simulink model "quad_simulation_with_linearization_around_wrench"  (R2018b)
settings: Solver=ode45  StartTime=0.0  StopTime=30  FixedStep=0.001  MaxStep=0.001  MinStep=0.0001  RelTol=1e-3
values from neighbouring files (symbols this model uses):
  b = 7e-9    (= 7e-09)    [Controller_Calc_W.m]    (also in Controller_Calc_Wrench.m; SDFO.m = parameters(7); SDR.m = parameters(7); hjb_minimum_fuel_continuous_time.m = parameters(7))
  g = 9.8    [Controller_Calc_W.m]    (also in Controller_Calc_Wrench.m; SDFO.m = parameters(12); SDR.m = parameters(12); hjb_minimum_fuel_continuous_time.m = parameters(12))
  Ixx = 2.661e-5    (= 2.661e-05)    [Controller_Calc_W.m]    (also in Controller_Calc_Wrench.m; SDFO.m = parameters(2); SDR.m = parameters(2); hjb_minimum_fuel_continuous_time.m = parameters(2))
  Iyy = 2.661e-5    (= 2.661e-05)    [Controller_Calc_W.m]    (also in Controller_Calc_Wrench.m; SDFO.m = parameters(3); SDR.m = parameters(3); hjb_minimum_fuel_continuous_time.m = parameters(3))
  Izz = 2.661e-5    (= 2.661e-05)    [Controller_Calc_W.m]    (also in Controller_Calc_Wrench.m; SDFO.m = parameters(4); SDR.m = parameters(4); hjb_minimum_fuel_continuous_time.m = parameters(4))
  k = 2e-6    (= 2e-06)    [Controller_Calc_W.m]    (also in Controller_Calc_Wrench.m; SDFO.m = parameters(5); SDR.m = parameters(5); hjb_minimum_fuel_continuous_time.m = parameters(5))
  K = zeros(4, 12, N)    [hjb_minimum_fuel_continuous_time.m]    (also in hjb_minimum_fuel_discrete_time.m)
  kd = 0    [Controller_Calc_W.m]    (also in Controller_Calc_Wrench.m; SDFO.m = parameters(8); SDR.m = parameters(8); hjb_minimum_fuel_continuous_time.m = parameters(8))
  L = 0.035    [Controller_Calc_W.m]    (also in Controller_Calc_Wrench.m; SDFO.m = parameters(6); SDR.m = parameters(6); hjb_minimum_fuel_continuous_time.m = parameters(6))
  m = w .* sign(w)    [SDFO.m]    (also in SDR.m = (u + ones(4, 1) * mq * g / 4); hjb_regulation_continuous_time.m = (u(:, i) + ones(4, 1) * mq * g / 4); hjb_regulation_discrete_time.m = (u(:, i) + ones(4, 1) * mq * g / 4))
  mq = 0.3812    [Controller_Calc_W.m]    (also in Controller_Calc_Wrench.m; SDFO.m = parameters(1); SDR.m = parameters(1); hjb_minimum_fuel_continuous_time.m = parameters(1))
  N = numel(t)    [Controller_Calc_W.m]    (also in Controller_Calc_Wrench.m; SDFO.m; SDR.m; hjb_minimum_fuel_continuous_time.m)
  r = 0.03    [Controller_Calc_W.m]    (also in Controller_Calc_Wrench.m; SDFO.m = parameters(10); SDR.m = parameters(10); hjb_minimum_fuel_continuous_time.m = parameters(10))
  rho = 0.037    [Controller_Calc_W.m]    (also in Controller_Calc_Wrench.m; SDFO.m = parameters(9); SDR.m = parameters(9); hjb_minimum_fuel_continuous_time.m = parameters(9))
  xd = 2    [Controller_Calc_W.m]    (also in Controller_Calc_Wrench.m; SDFO.m; SDR.m; hjb_minimum_fuel_continuous_time.m)
  yd = 2    [Controller_Calc_W.m]    (also in Controller_Calc_Wrench.m; SDFO.m; SDR.m; hjb_minimum_fuel_continuous_time.m)
  z_offset = 0.02    [Controller_Calc_W.m]    (also in Controller_Calc_Wrench.m; SDFO.m = parameters(11); SDR.m = parameters(11); hjb_minimum_fuel_continuous_time.m = parameters(11))
  zd = 1    [Controller_Calc_W.m]    (also in Controller_Calc_Wrench.m; SDFO.m; SDR.m; hjb_minimum_fuel_continuous_time.m)
undefined symbols (not defined in the file or in its folder): X, Y, Z
libraries: sm_lib x31, nesl_utility x15
settings Model: Creator=farid  LastModifiedBy=farid
settings SolverCC: ShapePreserveControl=EnableAll
settings DebuggingCC: IgnoredZcDiagnostic=none
settings ExplorerConfigSet: InternalSimMechanicsExplorerSettings="<ExplorerConfiguration><canonicalview>default</canonicalview><AnimationSetting><BasePlaybackSpeed>1.0</BasePlaybackSpeed><PlaybackSpeedFactor>1.0</PlaybackSpeedFactor></AnimationSetting><TilePanel><TileInfo><Tiles Columns=\"1\" Count=\"1\" Rows=\"1\"><Column Weight=\"1\"/><Row Weight=\"1\"/><Tile Height=\"1\" Width=\"1\" X=\"0\" Y=\"0\"/></Tiles></TileInfo><SceneInfo><SceneViewer><BGColor><R>0.60000002384185791</R><G>0.60000002384185791</G><B>0.60000002384185791</B></BGColor><Camera><DoPerspective>on</DoPerspective><Position><X>3.33949980158925674</X><Y>0.311821910931282698</Y><Z>2.70298018653747674</Z></Position><Center><X>1.08899615373952652</X><Y>1.13154056192934438</Y><Z>1.11569979798405505</Z></Center><Up><X>-0.544111387688414605</X><Y>0.115372635576885818</Y><Z>0.831042690087477443</Z></Up><ViewLimDist>1</ViewLimDist><YLim>0.466307658154998583</YLim><XLim>0.669757770788069529</XLim></Camera></SceneViewer></SceneInfo></TilePanel><MechEditorPanel><Cameras><Camera><Id>Camera1</Id><Value><Name>Camera1</Name><NativeCamera><PositionKeyframeSet/><CenterKeyframeSet/><UpVectorKeyframeSet/></NativeCamera></Value></Camera></Cameras><GfxPanelCameraMap><MapElement CameraMLId=\"Camera1\" GfxPanelIndex=\"0\"/></GfxPanelCameraMap><VideoCreator><PlaybackSpeedRatio>1.0</PlaybackSpeedRatio><FrameRate>60</FrameRate><VideoFormat>Motion JPEG AVI</VideoFormat><FrameSize>[1280 720]</FrameSize></VideoCreator></MechEditorPanel></ExplorerConfiguration>"

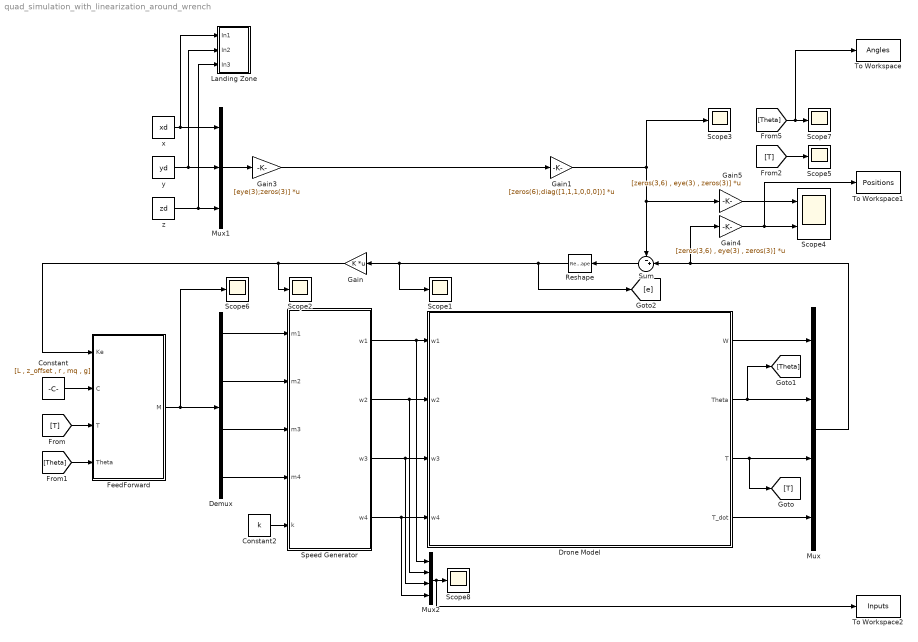
== system quad_simulation_with_linearization_around_wrench ==
  Constant : Constant  Value=[L , z_offset , r , mq , g]
  Constant2 : Constant  Value=k
  Demux : Demux
  Drone Model : Subsystem  mask{mq=mq, Ixx=Ixx, Iyy=Iyy, Izz=Izz, k=k, L=L, b=b, kd=kd, rho=rho, r=r, z_offset=z_offset, g=g}
      mask prompts: z_offset "offset in z:"
  FeedForward : MATLAB Function  TreatAsAtomicUnit=on
  Gain : Gain  Gain=K  Multiplication=Matrix(K*u) (u vector)
  Gain1 : Gain  Gain=[zeros(6);diag([1,1,1,0,0,0])]  Multiplication=Matrix(K*u) (u vector)
  Gain3 : Gain  Gain=[eye(3);zeros(3)]  Multiplication=Matrix(K*u) (u vector)
  Gain4 : Gain  Gain=[zeros(3,6) , eye(3) , zeros(3)]  Multiplication=Matrix(K*u) (u vector)
  Gain5 : Gain  Gain=[zeros(3,6) , eye(3) , zeros(3)]  Multiplication=Matrix(K*u) (u vector)
  Landing Zone : Subsystem
  Mux : Mux
  Mux1 : Mux  Inputs=3
  Mux2 : Mux
  Reshape : Reshape  OutputDimensionality=Column vector (2-D)
  Scope{1..3,5..8} (7 alike) : Scope
  Scope4 : Scope  NumInputPorts=2
  Speed Generator : MATLAB Function  TreatAsAtomicUnit=on
  Sum : Sum  Inputs=-+|
  To Workspace : ToWorkspace  VariableName=Angles  SaveFormat=Timeseries  SampleTime=-1
  To Workspace1 : ToWorkspace  VariableName=Positions  SaveFormat=Timeseries  SampleTime=-1
  To Workspace2 : ToWorkspace  VariableName=Inputs  SaveFormat=Timeseries  SampleTime=-1
  x : Constant  Value=xd
  y : Constant  Value=yd
  z : Constant  Value=zd
  wires:
  Speed Generator/1(w1) -> Mux2/1, Drone Model/1(w1)
  Speed Generator/2(w2) -> Mux2/2, Drone Model/2(w2)
  Speed Generator/3(w3) -> Mux2/3, Drone Model/3(w3)
  Speed Generator/4(w4) -> Mux2/4, Drone Model/4(w4)
  Drone Model/1(W) -> Mux/1
  Drone Model/2(Theta) -> [Theta], Mux/2
  Drone Model/3(T) -> [T], Mux/3
  Drone Model/4(T_dot) -> Mux/4
  Demux/1 -> Speed Generator/1(m1)
  Demux/2 -> Speed Generator/2(m2)
  Demux/3 -> Speed Generator/3(m3)
  Demux/4 -> Speed Generator/4(m4)
  Mux1/1 -> Gain3/1
  Mux/1 -> Gain4/1, Sum/2
  Gain3/1 -> Gain1/1
  Gain5/1 -> Scope4/1
  Gain4/1 -> To Workspace1/1, Scope4/2
  Gain1/1 -> Sum/1, Gain5/1, Scope3/1
  x/1 -> Landing Zone/1(In1), Mux1/1
  z/1 -> Landing Zone/3(In3), Mux1/3
  y/1 -> Landing Zone/2(In2), Mux1/2
  FeedForward/1(M) -> Scope6/1, Demux/1
  [T] -> FeedForward/3(T)
  [Theta] -> FeedForward/4(Theta)
  Constant/1 -> FeedForward/2(C)
  Sum/1 -> Reshape/1
  Reshape/1 -> [e], Gain/1, Scope1/1
  Gain/1 -> FeedForward/1(Ke), Scope2/1
  Constant2/1 -> Speed Generator/5(k)
  [Theta] -> To Workspace/1, Scope7/1
  [T] -> Scope5/1
  Mux2/1 -> To Workspace2/1, Scope8/1

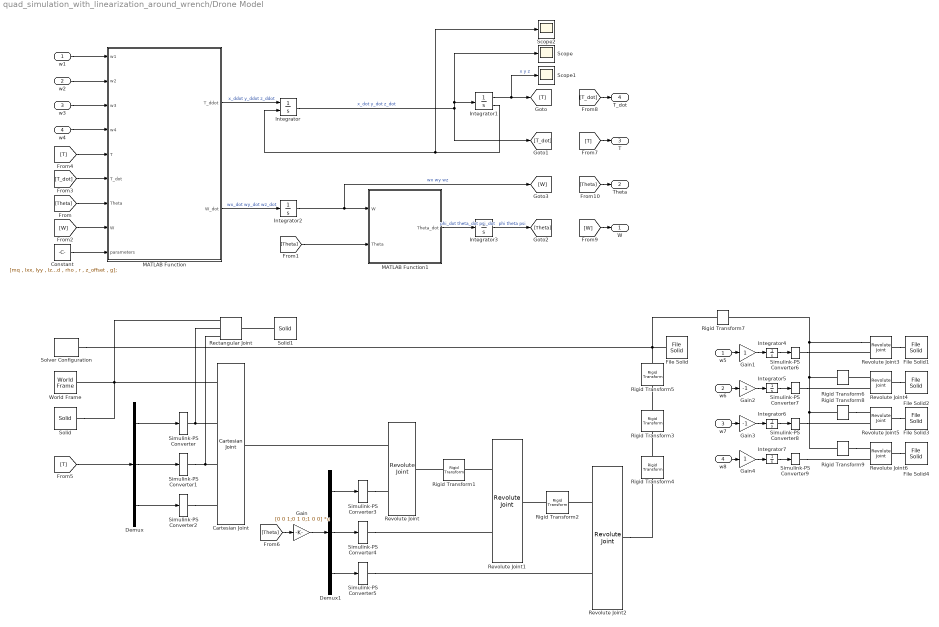
== system quad_simulation_with_linearization_around_wrench/Drone Model ==
  w1 : Inport
  w2 : Inport  Port=2
  w3 : Inport  Port=3
  w4 : Inport  Port=4
  Cartesian Joint : sm_lib/Joints/Cartesian Joint  SenseConstraintForce=off  SenseConstraintForceX=off  SenseConstraintForceY=off  SenseConstraintForceZ=off  SenseConstraintTorque=off  SenseConstraintTorqueX=off  SenseConstraintTorqueY=off  SenseConstraintTorqueZ=off  SenseTotalForce=off  SenseTotalForceX=off  SenseTotalForceY=off  SenseTotalForceZ=off  SenseTotalTorque=off  SenseTotalTorqueX=off  SenseTotalTorqueY=off  SenseTotalTorqueZ=off  CompositeWrenchDir=FollowerOnBase  CompositeWrenchFrame=BaseFrame  PxEquilibriumPosition=0  PxEquilibriumPositionUnits=m  PxSpringStiffness=0  PxSpringStiffnessUnits=N/m  PxDampingCoefficient=0  PxDampingCoefficientUnits=N/(m/s)  PxTorqueActuationMode=ComputedTorque  PxMotionActuationMode=InputMotion  PxSensePosition=off  PxSenseVelocity=off  PxSenseAcceleration=off  PxSenseTorqueForce=off  PxPositionTargetSpecify=off  PxPositionTargetPriority=High  PxPositionTargetValue=0  PxPositionTargetValueUnits=m  PxVelocityTargetSpecify=off  PxVelocityTargetPriority=High  PxVelocityTargetValue=0  PxVelocityTargetValueUnits=m/s  PyEquilibriumPosition=0  PyEquilibriumPositionUnits=m  PySpringStiffness=0  PySpringStiffnessUnits=N/m  PyDampingCoefficient=0  PyDampingCoefficientUnits=N/(m/s)  PyTorqueActuationMode=ComputedTorque  PyMotionActuationMode=InputMotion  PySensePosition=off  PySenseVelocity=off  PySenseAcceleration=off  PySenseTorqueForce=off  PyPositionTargetSpecify=off  PyPositionTargetPriority=High  PyPositionTargetValue=0  PyPositionTargetValueUnits=m  PyVelocityTargetSpecify=off  PyVelocityTargetPriority=High  PyVelocityTargetValue=0  PyVelocityTargetValueUnits=m/s  PzEquilibriumPosition=0  PzEquilibriumPositionUnits=m  PzSpringStiffness=0  PzSpringStiffnessUnits=N/m  PzDampingCoefficient=0  PzDampingCoefficientUnits=N/(m/s)  PzTorqueActuationMode=ComputedTorque  PzMotionActuationMode=InputMotion  PzSensePosition=off  PzSenseVelocity=off  PzSenseAcceleration=off  PzSenseTorqueForce=off  PzPositionTargetSpecify=on  PzPositionTargetPriority=High  PzPositionTargetValue=1  PzPositionTargetValueUnits=m  PzVelocityTargetSpecify=off  PzVelocityTargetPriority=High  PzVelocityTargetValue=0  PzVelocityTargetValueUnits=m/s
  Constant : Constant  Value=[mq , Ixx, Iyy , Izz , k , L , b , kd , rho , r , z_offset , g];
  Demux : Demux  Outputs=3
  Demux1 : Demux  Outputs=3
  File Solid : sm_lib/Body Elements/File Solid  ExtGeomFileName=/mnt/HDD Disk/Documents/MATLAB/Sahar Nasimi Nejad/dron.stl  UnitType=Custom  ExtGeomFileUnits=mm  InertiaType=Custom  Mass=1  MassUnits=kg  CenterOfMass=[0 0 0]  CenterOfMassUnits=m  MomentsOfInertia=[1 1 1]  MomentsOfInertiaUnits=kg*m^2  ProductsOfInertia=[0 0 0]  ProductsOfInertiaUnits=kg*m^2  BasedOnType=Density  Density=2  DensityUnits=g/cm^3  DoExposeReferenceFrame=on  SerializedFrames=<Frames/>  GraphicType=FromGeometry  MarkerShape=Sphere  MarkerSize=10  GraphicVisPropType=SimpleVisualProperties  GraphicDiffuseColor=[0.2 0.8 0.0]  GraphicSpecularColor=[0.5 0.5 0.5 1.0]  GraphicAmbientColor=[0.15 0.15 0.15 1.0]  GraphicEmissiveColor=[0.0 0.0 0.0 1.0]  GraphicShininess=75  GraphicOpacity=1.0
  File Solid{1..4} (4 alike) : sm_lib/Body Elements/File Solid  ExtGeomFileName=/mnt/HDD Disk/Documents/MATLAB/Optimal Control/propeller.stl  UnitType=Custom  ExtGeomFileUnits=mm  InertiaType=Custom  Mass=1  MassUnits=kg  CenterOfMass=[0 0 0]  CenterOfMassUnits=m  MomentsOfInertia=[1 1 1]  MomentsOfInertiaUnits=kg*m^2  ProductsOfInertia=[0 0 0]  ProductsOfInertiaUnits=kg*m^2  BasedOnType=Density  Density=2  DensityUnits=g/cm^3  DoExposeReferenceFrame=on  SerializedFrames=<Frames/>  GraphicType=FromGeometry  MarkerShape=Sphere  MarkerSize=10  GraphicVisPropType=SimpleVisualProperties  GraphicDiffuseColor=[1.0 1.0 0.0]  GraphicSpecularColor=[0.5 0.5 0.5 1.0]  GraphicAmbientColor=[0.15 0.15 0.15 1.0]  GraphicEmissiveColor=[0.0 0.0 0.0 1.0]  GraphicShininess=75  GraphicOpacity=1.0
  Gain : Gain  Gain=[0 0 1;0 1 0;1 0 0]  Multiplication=Matrix(K*u)
  Gain1 : Gain
  Gain2 : Gain  Gain=-1
  Gain3 : Gain  Gain=-1
  Gain4 : Gain
  Integrator : Integrator  ExternalReset=either  InitialCondition=[0;0;0]
  Integrator1 : Integrator  InitialCondition=[0;0;1]  LimitOutput=on  UpperSaturationLimit=[inf;inf;inf]  LowerSaturationLimit=[-inf;-inf;0]  ShowSaturationPort=on
  Integrator2 : Integrator  InitialCondition=[0;0;0]
  Integrator3 : Integrator  InitialCondition=[0;0;0]
  Integrator{4..7} (4 alike) : Integrator
  MATLAB Function : MATLAB Function  TreatAsAtomicUnit=on
  MATLAB Function1 : MATLAB Function  TreatAsAtomicUnit=on
  Rectangular Joint : sm_lib/Joints/Rectangular Joint  SenseConstraintForce=off  SenseConstraintForceX=off  SenseConstraintForceY=off  SenseConstraintForceZ=off  SenseConstraintTorque=off  SenseConstraintTorqueX=off  SenseConstraintTorqueY=off  SenseConstraintTorqueZ=off  SenseTotalForce=off  SenseTotalForceX=off  SenseTotalForceY=off  SenseTotalForceZ=off  SenseTotalTorque=off  SenseTotalTorqueX=off  SenseTotalTorqueY=off  SenseTotalTorqueZ=off  CompositeWrenchDir=FollowerOnBase  CompositeWrenchFrame=BaseFrame  PxEquilibriumPosition=0  PxEquilibriumPositionUnits=m  PxSpringStiffness=0  PxSpringStiffnessUnits=N/m  PxDampingCoefficient=0  PxDampingCoefficientUnits=N/(m/s)  PxTorqueActuationMode=ComputedTorque  PxMotionActuationMode=InputMotion  PxSensePosition=off  PxSenseVelocity=off  PxSenseAcceleration=off  PxSenseTorqueForce=off  PxPositionTargetSpecify=off  PxPositionTargetPriority=High  PxPositionTargetValue=0  PxPositionTargetValueUnits=m  PxVelocityTargetSpecify=off  PxVelocityTargetPriority=High  PxVelocityTargetValue=0  PxVelocityTargetValueUnits=m/s  PyEquilibriumPosition=0  PyEquilibriumPositionUnits=m  PySpringStiffness=0  PySpringStiffnessUnits=N/m  PyDampingCoefficient=0  PyDampingCoefficientUnits=N/(m/s)  PyTorqueActuationMode=ComputedTorque  PyMotionActuationMode=InputMotion  PySensePosition=off  PySenseVelocity=off  PySenseAcceleration=off  PySenseTorqueForce=off  PyPositionTargetSpecify=off  PyPositionTargetPriority=High  PyPositionTargetValue=0  PyPositionTargetValueUnits=m  PyVelocityTargetSpecify=off  PyVelocityTargetPriority=High  PyVelocityTargetValue=0  PyVelocityTargetValueUnits=m/s
      settings: SourceProductName=Simscape Multibody
  Revolute Joint{,1..6} (7 alike) : sm_lib/Joints/Revolute Joint  SenseConstraintForce=off  SenseConstraintForceX=off  SenseConstraintForceY=off  SenseConstraintForceZ=off  SenseConstraintTorque=off  SenseConstraintTorqueX=off  SenseConstraintTorqueY=off  SenseConstraintTorqueZ=off  SenseTotalForce=off  SenseTotalForceX=off  SenseTotalForceY=off  SenseTotalForceZ=off  SenseTotalTorque=off  SenseTotalTorqueX=off  SenseTotalTorqueY=off  SenseTotalTorqueZ=off  CompositeWrenchDir=FollowerOnBase  CompositeWrenchFrame=BaseFrame  EquilibriumPosition=0  EquilibriumPositionUnits=deg  SpringStiffness=0  SpringStiffnessUnits=N*m/deg  DampingCoefficient=0  DampingCoefficientUnits=N*m/(deg/s)  TorqueActuationMode=ComputedTorque  MotionActuationMode=InputMotion  SensePosition=off  SenseVelocity=off  SenseAcceleration=off  SenseTorqueForce=off  PositionTargetSpecify=off  PositionTargetPriority=High  PositionTargetValue=0  PositionTargetValueUnits=deg  VelocityTargetSpecify=off  VelocityTargetPriority=High  VelocityTargetValue=0  VelocityTargetValueUnits=deg/s
  Rigid Transform1 : sm_lib/Frames and Transforms/Rigid Transform  TranslationMethod=None  TranslationStandardOffset=0  TranslationLengthUnit=m  TranslationStandardAxis=+Z  TranslationCartesianOffset=[0 0 0]  TranslationROffset=0  TranslationROffsetUnits=m  TranslationZOffset=0  TranslationZOffsetUnits=m  TranslationThetaOffset=0  TranslationThetaOffsetUnits=deg  RotationMethod=StandardAxis  RotationAngleUnits=deg  RotationStandardAxis=-X  RotationAngle=90  RotationArbitraryAxis=[0 0 1]  FollAlignAxisA=+X  BaseAlignAxisA=+Y  FollAlignAxisB=+Y  BaseAlignAxisB=+Z  RotationSequenceAxes=FollowerAxes  RotationSequence=XYX  RotationSequenceAngles=[0 0 0]  RotationSequenceAnglesUnits=deg  RotationMatrix=[1 0 0; 0 1 0; 0 0 1]
  Rigid Transform2 : sm_lib/Frames and Transforms/Rigid Transform  TranslationMethod=None  TranslationStandardOffset=0  TranslationLengthUnit=m  TranslationStandardAxis=+Z  TranslationCartesianOffset=[0 0 0]  TranslationROffset=0  TranslationROffsetUnits=m  TranslationZOffset=0  TranslationZOffsetUnits=m  TranslationThetaOffset=0  TranslationThetaOffsetUnits=deg  RotationMethod=StandardAxis  RotationAngleUnits=deg  RotationStandardAxis=+Y  RotationAngle=90  RotationArbitraryAxis=[0 0 1]  FollAlignAxisA=+X  BaseAlignAxisA=+Y  FollAlignAxisB=+Y  BaseAlignAxisB=+Z  RotationSequenceAxes=FollowerAxes  RotationSequence=XYX  RotationSequenceAngles=[0 0 0]  RotationSequenceAnglesUnits=deg  RotationMatrix=[1 0 0; 0 1 0; 0 0 1]
  Rigid Transform3 : sm_lib/Frames and Transforms/Rigid Transform  TranslationMethod=None  TranslationStandardOffset=0  TranslationLengthUnit=m  TranslationStandardAxis=+Z  TranslationCartesianOffset=[0 0 0]  TranslationROffset=0  TranslationROffsetUnits=m  TranslationZOffset=0  TranslationZOffsetUnits=m  TranslationThetaOffset=0  TranslationThetaOffsetUnits=deg  RotationMethod=StandardAxis  RotationAngleUnits=deg  RotationStandardAxis=+X  RotationAngle=90  RotationArbitraryAxis=[0 0 1]  FollAlignAxisA=+X  BaseAlignAxisA=+Y  FollAlignAxisB=+Y  BaseAlignAxisB=+Z  RotationSequenceAxes=FollowerAxes  RotationSequence=XYX  RotationSequenceAngles=[0 0 0]  RotationSequenceAnglesUnits=deg  RotationMatrix=[1 0 0; 0 1 0; 0 0 1]
  Rigid Transform4 : sm_lib/Frames and Transforms/Rigid Transform  TranslationMethod=None  TranslationStandardOffset=0  TranslationLengthUnit=m  TranslationStandardAxis=+Z  TranslationCartesianOffset=[0 0 0]  TranslationROffset=0  TranslationROffsetUnits=m  TranslationZOffset=0  TranslationZOffsetUnits=m  TranslationThetaOffset=0  TranslationThetaOffsetUnits=deg  RotationMethod=StandardAxis  RotationAngleUnits=deg  RotationStandardAxis=-Y  RotationAngle=90  RotationArbitraryAxis=[0 0 1]  FollAlignAxisA=+X  BaseAlignAxisA=+Y  FollAlignAxisB=+Y  BaseAlignAxisB=+Z  RotationSequenceAxes=FollowerAxes  RotationSequence=XYX  RotationSequenceAngles=[0 0 0]  RotationSequenceAnglesUnits=deg  RotationMatrix=[1 0 0; 0 1 0; 0 0 1]
  Rigid Transform5 : sm_lib/Frames and Transforms/Rigid Transform  TranslationMethod=StandardAxis  TranslationStandardOffset=240  TranslationLengthUnit=mm  TranslationStandardAxis=+Z  TranslationCartesianOffset=[0 0 0]  TranslationROffset=0  TranslationROffsetUnits=m  TranslationZOffset=0  TranslationZOffsetUnits=m  TranslationThetaOffset=0  TranslationThetaOffsetUnits=deg  RotationMethod=StandardAxis  RotationAngleUnits=deg  RotationStandardAxis=+Z  RotationAngle=45  RotationArbitraryAxis=[0 0 1]  FollAlignAxisA=+X  BaseAlignAxisA=+Y  FollAlignAxisB=+Y  BaseAlignAxisB=+Z  RotationSequenceAxes=FollowerAxes  RotationSequence=XYX  RotationSequenceAngles=[0 0 0]  RotationSequenceAnglesUnits=deg  RotationMatrix=[1 0 0; 0 1 0; 0 0 1]
  Rigid Transform6 : sm_lib/Frames and Transforms/Rigid Transform  TranslationMethod=Cartesian  TranslationStandardOffset=0  TranslationLengthUnit=mm  TranslationStandardAxis=+Z  TranslationCartesianOffset=[-388.91 0 0]  TranslationROffset=0  TranslationROffsetUnits=m  TranslationZOffset=0  TranslationZOffsetUnits=m  TranslationThetaOffset=0  TranslationThetaOffsetUnits=deg  RotationMethod=None  RotationAngleUnits=deg  RotationStandardAxis=+Y  RotationAngle=90  RotationArbitraryAxis=[0 0 1]  FollAlignAxisA=+X  BaseAlignAxisA=+Y  FollAlignAxisB=+Y  BaseAlignAxisB=+Z  RotationSequenceAxes=FollowerAxes  RotationSequence=XYX  RotationSequenceAngles=[0 0 0]  RotationSequenceAnglesUnits=deg  RotationMatrix=[1 0 0; 0 1 0; 0 0 1]
  Rigid Transform7 : sm_lib/Frames and Transforms/Rigid Transform  TranslationMethod=Cartesian  TranslationStandardOffset=0  TranslationLengthUnit=mm  TranslationStandardAxis=+Z  TranslationCartesianOffset=[189.5 165.5 5]  TranslationROffset=0  TranslationROffsetUnits=m  TranslationZOffset=0  TranslationZOffsetUnits=m  TranslationThetaOffset=0  TranslationThetaOffsetUnits=deg  RotationMethod=None  RotationAngleUnits=deg  RotationStandardAxis=+Y  RotationAngle=90  RotationArbitraryAxis=[0 0 1]  FollAlignAxisA=+X  BaseAlignAxisA=+Y  FollAlignAxisB=+Y  BaseAlignAxisB=+Z  RotationSequenceAxes=FollowerAxes  RotationSequence=XYX  RotationSequenceAngles=[0 0 0]  RotationSequenceAnglesUnits=deg  RotationMatrix=[1 0 0; 0 1 0; 0 0 1]
  Rigid Transform8 : sm_lib/Frames and Transforms/Rigid Transform  TranslationMethod=Cartesian  TranslationStandardOffset=0  TranslationLengthUnit=mm  TranslationStandardAxis=+Z  TranslationCartesianOffset=[0 -388.9 0]  TranslationROffset=0  TranslationROffsetUnits=m  TranslationZOffset=0  TranslationZOffsetUnits=m  TranslationThetaOffset=0  TranslationThetaOffsetUnits=deg  RotationMethod=None  RotationAngleUnits=deg  RotationStandardAxis=+Y  RotationAngle=90  RotationArbitraryAxis=[0 0 1]  FollAlignAxisA=+X  BaseAlignAxisA=+Y  FollAlignAxisB=+Y  BaseAlignAxisB=+Z  RotationSequenceAxes=FollowerAxes  RotationSequence=XYX  RotationSequenceAngles=[0 0 0]  RotationSequenceAnglesUnits=deg  RotationMatrix=[1 0 0; 0 1 0; 0 0 1]
  Rigid Transform9 : sm_lib/Frames and Transforms/Rigid Transform  TranslationMethod=Cartesian  TranslationStandardOffset=0  TranslationLengthUnit=mm  TranslationStandardAxis=+Z  TranslationCartesianOffset=[-388.9 -388.9 0]  TranslationROffset=0  TranslationROffsetUnits=m  TranslationZOffset=0  TranslationZOffsetUnits=m  TranslationThetaOffset=0  TranslationThetaOffsetUnits=deg  RotationMethod=None  RotationAngleUnits=deg  RotationStandardAxis=+Y  RotationAngle=90  RotationArbitraryAxis=[0 0 1]  FollAlignAxisA=+X  BaseAlignAxisA=+Y  FollAlignAxisB=+Y  BaseAlignAxisB=+Z  RotationSequenceAxes=FollowerAxes  RotationSequence=XYX  RotationSequenceAngles=[0 0 0]  RotationSequenceAnglesUnits=deg  RotationMatrix=[1 0 0; 0 1 0; 0 0 1]
  Scope : Scope
  Scope1 : Scope
  Scope2 : Scope
  Simulink-PS Converter : nesl_utility/Simulink-PS Converter  PhysicalDomain=network_engine_domain  SubClassName=ps_input  LeftPortType=input  RightPortType=output  PseudoPeriodic=off  Frequencies=[]  NoiseDistribution=none  NoiseParameters=[]  Unit=1  AffineConversion=off  FilteringAndDerivatives=filter  SimscapeFilterOrder=2  InputFilterTimeConstant=0.001  UdotUserProvided=2
  Simulink-PS Converter1 : nesl_utility/Simulink-PS Converter  PhysicalDomain=network_engine_domain  SubClassName=ps_input  LeftPortType=input  RightPortType=output  PseudoPeriodic=off  Frequencies=[]  NoiseDistribution=none  NoiseParameters=[]  Unit=1  AffineConversion=off  FilteringAndDerivatives=filter  SimscapeFilterOrder=2  InputFilterTimeConstant=0.001  UdotUserProvided=2
  Simulink-PS Converter2 : nesl_utility/Simulink-PS Converter  PhysicalDomain=network_engine_domain  SubClassName=ps_input  LeftPortType=input  RightPortType=output  PseudoPeriodic=off  Frequencies=[]  NoiseDistribution=none  NoiseParameters=[]  Unit=1  AffineConversion=off  FilteringAndDerivatives=filter  SimscapeFilterOrder=2  InputFilterTimeConstant=0.001  UdotUserProvided=2
  Simulink-PS Converter{3..9} (7 alike) : nesl_utility/Simulink-PS Converter  PhysicalDomain=network_engine_domain  SubClassName=ps_input  LeftPortType=input  RightPortType=output  PseudoPeriodic=off  Frequencies=[]  NoiseDistribution=none  NoiseParameters=[]  Unit=rad  AffineConversion=off  FilteringAndDerivatives=filter  SimscapeFilterOrder=2  InputFilterTimeConstant=0.001  UdotUserProvided=2
  Solid : sm_lib/Body Elements/Solid  InertiaType=CalculateFromGeometry  Mass=1  MassUnits=kg  CenterOfMass=[0 0 0]  CenterOfMassUnits=m  MomentsOfInertia=[1 1 1]  MomentsOfInertiaUnits=kg*m^2  ProductsOfInertia=[0 0 0]  ProductsOfInertiaUnits=kg*m^2  BasedOnType=Density  Density=1000  DensityUnits=kg/m^3  DoExposeReferenceFrame=on  SerializedFrames=<Frames/>  GraphicType=None  MarkerShape=Sphere  MarkerSize=10  GraphicVisPropType=SimpleVisualProperties  GraphicDiffuseColor=[0.0 0.0 0.4]  GraphicSpecularColor=[0.5 0.5 0.5 1.0]  GraphicAmbientColor=[0.15 0.15 0.15 1.0]  GraphicEmissiveColor=[0.0 0.0 0.0 1.0]  GraphicShininess=75  GraphicOpacity=1.0  GeometryShape=Brick  RectangleSize=[1 1]  RectangleSizeUnits=m  BrickDimensions=[10 10 0.095]  BrickDimensionUnits=m  CylinderRadius=1  CylinderRadiusUnits=m  CylinderLength=1  CylinderLengthUnits=m  SphereRadius=1  SphereRadiusUnits=m  EllipsoidRadii=[1 1 1]  EllipsoidRadiiUnits=m  ExtrusionCrossSection=[1 1; -1 1; -1 -1; 1 -1]  ExtrusionCrossSectionUnits=m  ExtrusionLength=1  ExtrusionLengthUnits=m  PolygonNumSides=3  PolygonOuterRadius=1  PolygonOuterRadiusUnits=m  ExtGeomFileType=STEP  ExtGeomFileUnits=m  RevolutionCrossSection=[1 1; 1 -1; 2 -1; 2 1]  RevolutionCrossSectionUnits=m  RevolutionExtent=Full  RevolutionAngle=180  RevolutionAngleUnits=deg
  Solid1 : sm_lib/Body Elements/Solid  InertiaType=CalculateFromGeometry  Mass=1  MassUnits=kg  CenterOfMass=[0 0 0]  CenterOfMassUnits=m  MomentsOfInertia=[1 1 1]  MomentsOfInertiaUnits=kg*m^2  ProductsOfInertia=[0 0 0]  ProductsOfInertiaUnits=kg*m^2  BasedOnType=Density  Density=1000  DensityUnits=kg/m^3  DoExposeReferenceFrame=on  SerializedFrames=<Frames/>  GraphicType=None  MarkerShape=Sphere  MarkerSize=10  GraphicVisPropType=SimpleVisualProperties  GraphicDiffuseColor=[0.4 1.0 0.0]  GraphicSpecularColor=[0.5 0.5 0.5 1.0]  GraphicAmbientColor=[0.15 0.15 0.15 1.0]  GraphicEmissiveColor=[0.0 0.0 0.0 1.0]  GraphicShininess=75  GraphicOpacity=0.3  GeometryShape=Cylinder  RectangleSize=[1 1]  RectangleSizeUnits=m  BrickDimensions=[0.1 0.1 0.1]  BrickDimensionUnits=m  CylinderRadius=0.5  CylinderRadiusUnits=m  CylinderLength=0.15  CylinderLengthUnits=m  SphereRadius=1  SphereRadiusUnits=m  EllipsoidRadii=[1 1 1]  EllipsoidRadiiUnits=m  ExtrusionCrossSection=[1 1; -1 1; -1 -1; 1 -1]  ExtrusionCrossSectionUnits=m  ExtrusionLength=1  ExtrusionLengthUnits=m  PolygonNumSides=3  PolygonOuterRadius=1  PolygonOuterRadiusUnits=m  ExtGeomFileType=STEP  ExtGeomFileUnits=m  RevolutionCrossSection=[1 1; 1 -1; 2 -1; 2 1]  RevolutionCrossSectionUnits=m  RevolutionExtent=Full  RevolutionAngle=180  RevolutionAngleUnits=deg
  Solver Configuration : nesl_utility/Solver Configuration  PhysicalDomain=network_engine_domain  SubClassName=solver  LeftPortType=input  RightPortType=generic  Tones=[]  Harmonics=[]  SimulateNoise=off  Profile=off  UseLocalSampling=off  EnableSwitchedLinearOptims=on  FrequencyDomain=off  UseCCode=off  RelTol=0.001  AbsTol=1e-06  MinStep=1e-09  ToWorkspace=off  RevertToSquareIcSolve=off  NumHomotopyIterations=100  PhasorMode=off  PhasorModeNumHarmonics=1  DoDC=off  ResidualTolerance=1e-09  UseLocalSolver=off  LocalSolverChoice=NE_BACKWARD_EULER_ADVANCER  LocalSolverSampleTime=0.001  DoFixedCost=off  MaxNonlinIter=3  MaxModeIter=2  LinearAlgebra=auto  EquationFormulation=NE_TIME_EF  DelaysMemoryBudget=1024  AutomaticFiltering=on  FilteringTimeConstant=0.0001  PartitionStorageMethod=AS_NEEDED  PartitionMemoryBudget=1024
  World Frame : sm_lib/Frames and Transforms/World Frame
  w5 : InportShadow
  w6 : InportShadow  Port=2
  w7 : InportShadow  Port=3
  w8 : InportShadow  Port=4
  W : Outport
  Theta : Outport  Port=2
  T : Outport  Port=3
  T_dot : Outport  Port=4
  wires:
  MATLAB Function/1(T_ddot) -> Integrator/1  "x_ddot y_ddot z_ddot"
  [Theta] -> Theta/1
  [T_dot] -> MATLAB Function/6(T_dot)
  [W] -> MATLAB Function/8(W)
  Constant/1 -> MATLAB Function/9(parameters)
  [T] -> Demux/1
  [Theta] -> MATLAB Function1/2(Theta)
  [T] -> MATLAB Function/5(T)
  Integrator1/1 -> Scope1/1, [T]  "x y z"
  w4/1 -> MATLAB Function/4(w4)
  w2/1 -> MATLAB Function/2(w2)
  [T_dot] -> T_dot/1
  Demux/1 -> Simulink-PS Converter/1
  Demux1/3 -> Simulink-PS Converter5/1
  [T] -> T/1
  Integrator2/1 -> [W], MATLAB Function1/1(W)  "wx wy wz"
  Demux1/2 -> Simulink-PS Converter4/1
  w1/1 -> MATLAB Function/1(w1)
  w3/1 -> MATLAB Function/3(w3)
  MATLAB Function/2(W_dot) -> Integrator2/1  "wx_dot wy_dot wz_dot"
  Demux1/1 -> Simulink-PS Converter3/1
  [W] -> W/1
  [Theta] -> MATLAB Function/7(Theta)
  Integrator3/1 -> [Theta]  "phi theta psi"
  [Theta] -> Gain/1
  Demux/3 -> Simulink-PS Converter2/1
  Integrator/1 -> Scope/1, Integrator1/1, [T_dot]  "x_dot y_dot z_dot"
  MATLAB Function1/1(Theta_dot) -> Integrator3/1  "phi_dot theta_dot psi_dot"
  Demux/2 -> Simulink-PS Converter1/1
  Gain/1 -> Demux1/1
  Integrator1/2 -> Scope2/1, Integrator/2
  Integrator4/1 -> Simulink-PS Converter6/1
  Integrator5/1 -> Simulink-PS Converter7/1
  Integrator6/1 -> Simulink-PS Converter8/1
  Integrator7/1 -> Simulink-PS Converter9/1
  w5/1 -> Gain1/1
  Gain1/1 -> Integrator4/1
  w6/1 -> Gain2/1
  Gain2/1 -> Integrator5/1
  w7/1 -> Gain3/1
  Gain3/1 -> Integrator6/1
  w8/1 -> Gain4/1
  Gain4/1 -> Integrator7/1
  connections:
  Rigid Transform4/RConn1 -- Rigid Transform3/LConn1
  Revolute Joint1/LConn1 -- Rigid Transform1/RConn1
  Revolute Joint2/RConn1 -- Rigid Transform4/LConn1
  Revolute Joint2/LConn1 -- Rigid Transform2/RConn1
  Cartesian Joint/LConn1 -- Solid/RConn1 -- Rectangular Joint/LConn1 -- World Frame/RConn1
  Simulink-PS Converter5/RConn1 -- Revolute Joint2/LConn2
  Simulink-PS Converter/RConn1 -- Rectangular Joint/LConn2 -- Cartesian Joint/LConn2
  Revolute Joint/LConn1 -- Cartesian Joint/RConn1
  Rigid Transform2/LConn1 -- Revolute Joint1/RConn1
  Simulink-PS Converter2/RConn1 -- Cartesian Joint/LConn4
  Simulink-PS Converter3/RConn1 -- Revolute Joint/LConn2
  Simulink-PS Converter1/RConn1 -- Rectangular Joint/LConn3 -- Cartesian Joint/LConn3
  Simulink-PS Converter4/RConn1 -- Revolute Joint1/LConn2
  Rigid Transform1/LConn1 -- Revolute Joint/RConn1
  Rigid Transform3/RConn1 -- Rigid Transform5/LConn1
  Revolute Joint3/RConn1 -- File Solid1/RConn1
  Revolute Joint4/RConn1 -- File Solid2/RConn1
  Revolute Joint5/RConn1 -- File Solid3/RConn1
  Revolute Joint6/RConn1 -- File Solid4/RConn1
  Revolute Joint4/LConn1 -- Rigid Transform6/RConn1
  Simulink-PS Converter6/RConn1 -- Revolute Joint3/LConn2
  Simulink-PS Converter7/RConn1 -- Revolute Joint4/LConn2
  Simulink-PS Converter8/RConn1 -- Revolute Joint5/LConn2
  Simulink-PS Converter9/RConn1 -- Revolute Joint6/LConn2
  Solver Configuration/RConn1 -- Rigid Transform7/LConn1 -- Rigid Transform5/RConn1 -- File Solid/RConn1
  Revolute Joint3/LConn1 -- Rigid Transform6/LConn1 -- Rigid Transform9/LConn1 -- Rigid Transform8/LConn1 -- Rigid Transform7/RConn1
  Rigid Transform8/RConn1 -- Revolute Joint5/LConn1
  Rigid Transform9/RConn1 -- Revolute Joint6/LConn1
  Solid1/RConn1 -- Rectangular Joint/RConn1

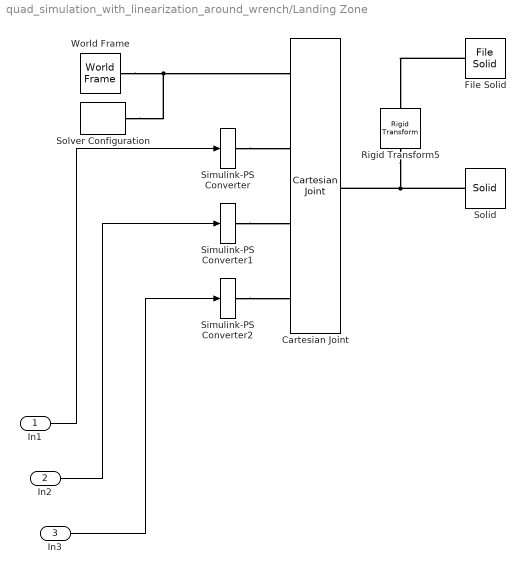
== system quad_simulation_with_linearization_around_wrench/Landing Zone ==
  In1 : Inport
  In2 : Inport  Port=2
  In3 : Inport  Port=3
  Cartesian Joint : sm_lib/Joints/Cartesian Joint  SenseConstraintForce=off  SenseConstraintForceX=off  SenseConstraintForceY=off  SenseConstraintForceZ=off  SenseConstraintTorque=off  SenseConstraintTorqueX=off  SenseConstraintTorqueY=off  SenseConstraintTorqueZ=off  SenseTotalForce=off  SenseTotalForceX=off  SenseTotalForceY=off  SenseTotalForceZ=off  SenseTotalTorque=off  SenseTotalTorqueX=off  SenseTotalTorqueY=off  SenseTotalTorqueZ=off  CompositeWrenchDir=FollowerOnBase  CompositeWrenchFrame=BaseFrame  PxEquilibriumPosition=0  PxEquilibriumPositionUnits=m  PxSpringStiffness=0  PxSpringStiffnessUnits=N/m  PxDampingCoefficient=0  PxDampingCoefficientUnits=N/(m/s)  PxTorqueActuationMode=ComputedTorque  PxMotionActuationMode=InputMotion  PxSensePosition=off  PxSenseVelocity=off  PxSenseAcceleration=off  PxSenseTorqueForce=off  PxPositionTargetSpecify=off  PxPositionTargetPriority=High  PxPositionTargetValue=0  PxPositionTargetValueUnits=m  PxVelocityTargetSpecify=off  PxVelocityTargetPriority=High  PxVelocityTargetValue=0  PxVelocityTargetValueUnits=m/s  PyEquilibriumPosition=0  PyEquilibriumPositionUnits=m  PySpringStiffness=0  PySpringStiffnessUnits=N/m  PyDampingCoefficient=0  PyDampingCoefficientUnits=N/(m/s)  PyTorqueActuationMode=ComputedTorque  PyMotionActuationMode=InputMotion  PySensePosition=off  PySenseVelocity=off  PySenseAcceleration=off  PySenseTorqueForce=off  PyPositionTargetSpecify=off  PyPositionTargetPriority=High  PyPositionTargetValue=0  PyPositionTargetValueUnits=m  PyVelocityTargetSpecify=off  PyVelocityTargetPriority=High  PyVelocityTargetValue=0  PyVelocityTargetValueUnits=m/s  PzEquilibriumPosition=0  PzEquilibriumPositionUnits=m  PzSpringStiffness=0  PzSpringStiffnessUnits=N/m  PzDampingCoefficient=0  PzDampingCoefficientUnits=N/(m/s)  PzTorqueActuationMode=ComputedTorque  PzMotionActuationMode=InputMotion  PzSensePosition=off  PzSenseVelocity=off  PzSenseAcceleration=off  PzSenseTorqueForce=off  PzPositionTargetSpecify=off  PzPositionTargetPriority=High  PzPositionTargetValue=0  PzPositionTargetValueUnits=m  PzVelocityTargetSpecify=off  PzVelocityTargetPriority=High  PzVelocityTargetValue=0  PzVelocityTargetValueUnits=m/s
  File Solid : sm_lib/Body Elements/File Solid  ExtGeomFileName=/mnt/HDD Disk/Documents/MATLAB/Sahar Nasimi Nejad/dron.stl  UnitType=Custom  ExtGeomFileUnits=mm  InertiaType=Custom  Mass=1  MassUnits=kg  CenterOfMass=[0 0 0]  CenterOfMassUnits=m  MomentsOfInertia=[1 1 1]  MomentsOfInertiaUnits=kg*m^2  ProductsOfInertia=[0 0 0]  ProductsOfInertiaUnits=kg*m^2  BasedOnType=Density  Density=2  DensityUnits=g/cm^3  DoExposeReferenceFrame=on  SerializedFrames=<Frames/>  GraphicType=FromGeometry  MarkerShape=Sphere  MarkerSize=10  GraphicVisPropType=SimpleVisualProperties  GraphicDiffuseColor=[1.0 0.0 0.0]  GraphicSpecularColor=[0.5 0.5 0.5 1.0]  GraphicAmbientColor=[0.15 0.15 0.15 1.0]  GraphicEmissiveColor=[0.0 0.0 0.0 1.0]  GraphicShininess=75  GraphicOpacity=0.4
  Rigid Transform5 : sm_lib/Frames and Transforms/Rigid Transform  TranslationMethod=StandardAxis  TranslationStandardOffset=240  TranslationLengthUnit=mm  TranslationStandardAxis=+Z  TranslationCartesianOffset=[0 0 0]  TranslationROffset=0  TranslationROffsetUnits=m  TranslationZOffset=0  TranslationZOffsetUnits=m  TranslationThetaOffset=0  TranslationThetaOffsetUnits=deg  RotationMethod=StandardAxis  RotationAngleUnits=deg  RotationStandardAxis=+Z  RotationAngle=45  RotationArbitraryAxis=[0 0 1]  FollAlignAxisA=+X  BaseAlignAxisA=+Y  FollAlignAxisB=+Y  BaseAlignAxisB=+Z  RotationSequenceAxes=FollowerAxes  RotationSequence=XYX  RotationSequenceAngles=[0 0 0]  RotationSequenceAnglesUnits=deg  RotationMatrix=[1 0 0; 0 1 0; 0 0 1]
  Simulink-PS Converter : nesl_utility/Simulink-PS Converter  PhysicalDomain=network_engine_domain  SubClassName=ps_input  LeftPortType=input  RightPortType=output  PseudoPeriodic=off  Frequencies=[]  NoiseDistribution=none  NoiseParameters=[]  Unit=1  AffineConversion=off  FilteringAndDerivatives=filter  SimscapeFilterOrder=2  InputFilterTimeConstant=0.001  UdotUserProvided=2
  Simulink-PS Converter1 : nesl_utility/Simulink-PS Converter  PhysicalDomain=network_engine_domain  SubClassName=ps_input  LeftPortType=input  RightPortType=output  PseudoPeriodic=off  Frequencies=[]  NoiseDistribution=none  NoiseParameters=[]  Unit=1  AffineConversion=off  FilteringAndDerivatives=filter  SimscapeFilterOrder=2  InputFilterTimeConstant=0.001  UdotUserProvided=2
  Simulink-PS Converter2 : nesl_utility/Simulink-PS Converter  PhysicalDomain=network_engine_domain  SubClassName=ps_input  LeftPortType=input  RightPortType=output  PseudoPeriodic=off  Frequencies=[]  NoiseDistribution=none  NoiseParameters=[]  Unit=1  AffineConversion=off  FilteringAndDerivatives=filter  SimscapeFilterOrder=2  InputFilterTimeConstant=0.001  UdotUserProvided=2
  Solid : sm_lib/Body Elements/Solid  InertiaType=CalculateFromGeometry  Mass=1  MassUnits=kg  CenterOfMass=[0 0 0]  CenterOfMassUnits=m  MomentsOfInertia=[1 1 1]  MomentsOfInertiaUnits=kg*m^2  ProductsOfInertia=[0 0 0]  ProductsOfInertiaUnits=kg*m^2  BasedOnType=Density  Density=1000  DensityUnits=kg/m^3  DoExposeReferenceFrame=on  SerializedFrames=<Frames/>  GraphicType=None  MarkerShape=Sphere  MarkerSize=10  GraphicVisPropType=SimpleVisualProperties  GraphicDiffuseColor=[1.0 0.0 0.2]  GraphicSpecularColor=[0.5 0.5 0.5 1.0]  GraphicAmbientColor=[0.15 0.15 0.15 1.0]  GraphicEmissiveColor=[0.0 0.0 0.0 1.0]  GraphicShininess=75  GraphicOpacity=1.0  GeometryShape=Cylinder  RectangleSize=[1 1]  RectangleSizeUnits=m  BrickDimensions=[0.1 0.1 0.1]  BrickDimensionUnits=m  CylinderRadius=0.5  CylinderRadiusUnits=m  CylinderLength=0.1  CylinderLengthUnits=m  SphereRadius=1  SphereRadiusUnits=m  EllipsoidRadii=[1 1 1]  EllipsoidRadiiUnits=m  ExtrusionCrossSection=[1 1; -1 1; -1 -1; 1 -1]  ExtrusionCrossSectionUnits=m  ExtrusionLength=1  ExtrusionLengthUnits=m  PolygonNumSides=3  PolygonOuterRadius=1  PolygonOuterRadiusUnits=m  ExtGeomFileType=STEP  ExtGeomFileUnits=m  RevolutionCrossSection=[1 1; 1 -1; 2 -1; 2 1]  RevolutionCrossSectionUnits=m  RevolutionExtent=Full  RevolutionAngle=180  RevolutionAngleUnits=deg
  Solver Configuration : nesl_utility/Solver Configuration  PhysicalDomain=network_engine_domain  SubClassName=solver  LeftPortType=input  RightPortType=generic  Tones=[]  Harmonics=[]  SimulateNoise=off  Profile=off  UseLocalSampling=off  EnableSwitchedLinearOptims=on  FrequencyDomain=off  UseCCode=off  RelTol=0.001  AbsTol=1e-06  MinStep=1e-09  ToWorkspace=off  RevertToSquareIcSolve=off  NumHomotopyIterations=100  PhasorMode=off  PhasorModeNumHarmonics=1  DoDC=off  ResidualTolerance=1e-09  UseLocalSolver=off  LocalSolverChoice=NE_BACKWARD_EULER_ADVANCER  LocalSolverSampleTime=0.001  DoFixedCost=off  MaxNonlinIter=3  MaxModeIter=2  LinearAlgebra=auto  EquationFormulation=NE_TIME_EF  DelaysMemoryBudget=1024  AutomaticFiltering=on  FilteringTimeConstant=0.0001  PartitionStorageMethod=AS_NEEDED  PartitionMemoryBudget=1024
  World Frame : sm_lib/Frames and Transforms/World Frame
  wires:
  In3/1 -> Simulink-PS Converter2/1
  In1/1 -> Simulink-PS Converter/1
  In2/1 -> Simulink-PS Converter1/1
  connections:
  Simulink-PS Converter/RConn1 -- Cartesian Joint/LConn2
  Simulink-PS Converter2/RConn1 -- Cartesian Joint/LConn4
  Simulink-PS Converter1/RConn1 -- Cartesian Joint/LConn3
  World Frame/RConn1 -- Solver Configuration/RConn1 -- Cartesian Joint/LConn1
  Solid/RConn1 -- Cartesian Joint/RConn1 -- Rigid Transform5/LConn1
  File Solid/RConn1 -- Rigid Transform5/RConn1

== matlab function quad_simulation_with_linearization_around_wrench/Drone Model/MATLAB Function1 ==
  data: W input; Theta_dot output; Theta input
function Theta_dot = fcn(W , Theta)

phi     = Theta(1);
theta   = Theta(2);
psi     = Theta(3);

E = [1 , sin(phi)*tan(theta) ,  cos(phi)*tan(theta);
     0 , cos(phi)            , -sin(phi)           ;
     0 , sin(phi)/cos(theta) , cos(phi)/cos(theta) ;];

Theta_dot = E*W;
end

== matlab function quad_simulation_with_linearization_around_wrench/Drone Model/MATLAB Function ==
  data: w1 input; T_ddot output; w2 input; w3 input; w4 input; T input; T_dot input; Theta input; W input; parameters input; W_dot output
function [T_ddot , W_dot] = fcn(w1 , w2 , w3 , w4 , T , T_dot , Theta , W , parameters)

%% parameters

mq = parameters(1);
Ixx = parameters(2);
Iyy = parameters(3);
Izz = parameters(4);
k = parameters(5);
L = parameters(6);
b = parameters(7);
kd = parameters(8);
rho = parameters(9);
r = parameters(10);
z_offset = parameters(11);
g = parameters(12);

%% states

x       = T(1);
y       = T(2);
z       = T(3);

phi     = Theta(1);
theta   = Theta(2);
psi     = Theta(3);

%% Matrices

Rx = [1 0 0;0 cos(phi) -sin(phi);0 sin(phi) cos(phi)];
Ry = [cos(theta) 0 sin(theta);0 1 0;-sin(theta) 0 cos(theta)];
Rz = [cos(psi) -sin(psi) 0;sin(psi) cos(psi) 0;0 0 1];
R = Rz*Ry*Rx;

I = diag([Ixx , Iyy , Izz]);


%% Input Modification

in = zeros(4,1);
Ground_Effect_Coef = @(z) 1;
z1 = [0 0 1]*([x;y;z] + R*[0;L;z_offset]);
z2 = [0 0 1]*([x;y;z] + R*[-L;0;z_offset]);
z3 = [0 0 1]*([x;y;z] + R*[0;-L;z_offset]);
z4 = [0 0 1]*([x;y;z] + R*[L;0;z_offset]);
in(1) = Ground_Effect_Coef(z1)*w1*abs(w1);
in(2) = Ground_Effect_Coef(z2)*w2*abs(w2);
in(3) = Ground_Effect_Coef(z3)*w3*abs(w3);
in(4) = Ground_Effect_Coef(z4)*w4*abs(w4);

%% Translational Dynamics

TB = k*[0;0;sum(in)];        %trust force with ground effect
FD = -kd*T_dot;             %frictional force
T_ddot = [0;0;-g] + (R*TB + FD)/mq;    %Translational Dynamics

%% Rotational Dynamics

tau = [L*k*(in(1) - in(3));L*k*(in(2)-in(4));b*(in(1)-in(2)+in(3)-in(4))]; %Rotational Torque with ground effect
W_dot = I\(tau - cross(W , I*W));                                          %Rotational Dynamics

end

== matlab function quad_simulation_with_linearization_around_wrench/Speed Generator ==
  data: m1 input; w1 output; m2 input; m3 input; m4 input; w2 output; w3 output; w4 output; k input
function [w1 , w2 , w3 , w4] = fcn(m1, m2 , m3 , m4 , k)

w1 = sign(m1)*(abs(m1/k)^0.5);
w2 = sign(m2)*(abs(m2/k)^0.5);
w3 = sign(m3)*(abs(m3/k)^0.5);
w4 = sign(m4)*(abs(m4/k)^0.5);

== matlab function quad_simulation_with_linearization_around_wrench/FeedForward ==
  data: Ke input; C input; T input; M output; Theta input
function M = fcn(Ke , C, T , Theta)

L = C(1);
z_offset = C(2);
r = C(3);
mq = C(4);
g = C(5);

x       = T(1);
y       = T(2);
z       = T(3);

phi     = Theta(1);
theta   = Theta(2);
psi     = Theta(3);

Rx = [1 0 0;0 cos(phi) -sin(phi);0 sin(phi) cos(phi)];
Ry = [cos(theta) 0 sin(theta);0 1 0;-sin(theta) 0 cos(theta)];
Rz = [cos(psi) -sin(psi) 0;sin(psi) cos(psi) 0;0 0 1];
R = Rz*Ry*Rx;

z1 = [0 0 1]*([x;y;z] + R*[0;L;z_offset]);
z2 = [0 0 1]*([x;y;z] + R*[-L;0;z_offset]);
z3 = [0 0 1]*([x;y;z] + R*[0;-L;z_offset]);
z4 = [0 0 1]*([x;y;z] + R*[L;0;z_offset]);

Ground_Effect_Coef = @(z) 1;

M = diag([1/Ground_Effect_Coef(z1),...
          1/Ground_Effect_Coef(z2),...
          1/Ground_Effect_Coef(z3),...
          1/Ground_Effect_Coef(z4)])*(-Ke + ones(4,1)*mq*g/4);
